simulink model "mod_integrador"  (R2020a)
settings: Solver=FixedStepAuto  StartTime=0.0  StopTime=t_fim  FixedStep=dt_sim  RelTol=1e-3
values from neighbouring files (symbols this model uses):
  Ac = [0, 1;0, 0]    [init.m]    (also in run.m = evalin('base', 'Ac'))
  Bc = [0; 1]    [init.m]    (also in run.m = evalin('base', 'Bc'))
  bf = aux(:,end)    [matrizes_ss_mpc_dualmode_switching.m]    (also in run.m = evalin('base', 'bf'))
  cbar = repmat(c,Np,1)    [matrizes_ss_mpc_dualmode_switching.m]    (also in run.m = evalin('base', 'cbar'))
  dt_sim = 0.001    [init.m]
  H = zeros(n*Np,p*Np)    [matrizes_ss_mpc_dualmode_switching.m]    (also in run.m = evalin('base', 'H'))
  Hf = H(end-n+1:end,:)    [matrizes_ss_mpc_dualmode_switching.m]    (also in run.m = evalin('base', 'Hf'))
  Lbar = blkdiag(Lbar,L)    [matrizes_ss_mpc_dualmode_switching.m]    (also in run.m = evalin('base', 'Lbar'))
  p = find(dt == 1, 2, 'last')    [get_xr.m]    (also in init.m = N - 1; matrizes_ss_mpc_dualmode_switching.m = size(Gamma,2); run.m = evalin('base', 'p'))
  Pf = dlyap(Phib',Phib'*Q*Phib + K'*R*K)    [matrizes_ss_mpc_dualmode_switching.m]    (also in run.m = evalin('base', 'Pf'))
  Phi1Np = [Phi1Np;Phi^i]    [matrizes_ss_mpc_dualmode_switching.m]    (also in run.m = evalin('base', 'Phi1Np'))
  PhiNp = Phi^Np    [matrizes_ss_mpc_dualmode_switching.m]    (also in run.m = evalin('base', 'PhiNp'))
  Qbar = blkdiag(Qbar,Q)    [matrizes_ss_mpc_dualmode_switching.m]    (also in run.m = evalin('base', 'Qbar'))
  Rbar = blkdiag(Rbar,R)    [matrizes_ss_mpc_dualmode_switching.m]    (also in run.m = evalin('base', 'Rbar'))
  Sf = aux(:,1:(end-1))    [matrizes_ss_mpc_dualmode_switching.m]    (also in run.m = evalin('base', 'Sf'))
  T = sum(dtr)    [init.m]
  tr = [2, 3, 5, 6]'    [init.m]    (also in run.m = evalin('base', 'tr'))
  ur = [1, 0, -1, 0]'    [init.m]    (also in run.m = evalin('base', 'ur'))
  x0 = [-0.5; -1]    [init.m]    (also in mpc_dualmode_switching.m = zeros(size(fqp, 1), 1); run.m = y_(end,:)')
  x_target = x0    [init.m]    (also in run.m)
settings Model: Creator=Daniel  LastModifiedBy=Daniel
settings DataIOCC: SaveOutput=off  DSMLogging=off  SaveTime=off

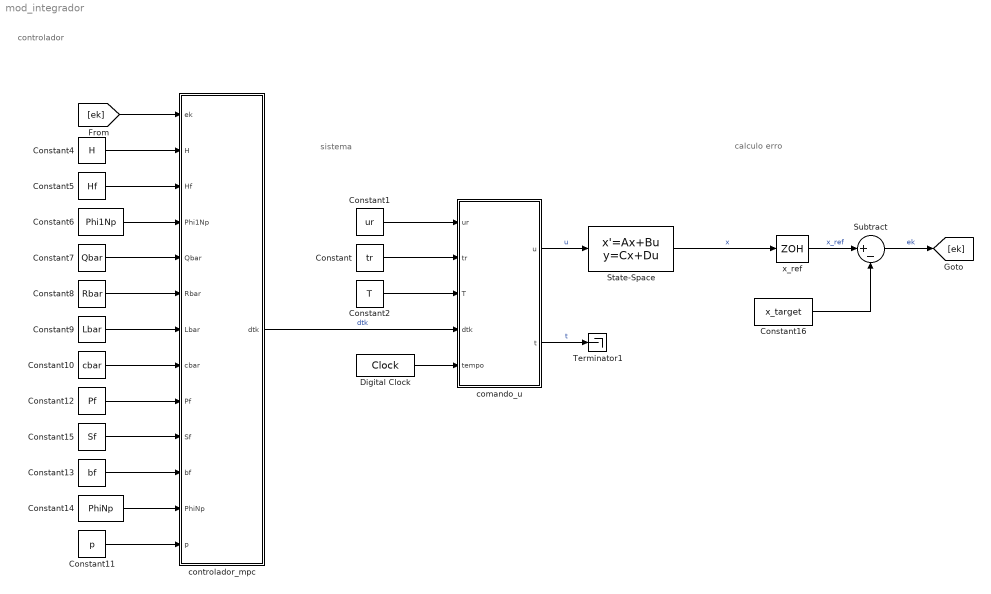
== system mod_integrador ==
  note: calculo erro
  note: controlador
  note: sistema
  Constant : Constant  Value=tr
  Constant1 : Constant  Value=ur
  Constant10 : Constant  Value=cbar
  Constant11 : Constant  Value=p
  Constant12 : Constant  Value=Pf
  Constant13 : Constant  Value=bf
  Constant14 : Constant  Value=PhiNp
  Constant15 : Constant  Value=Sf
  Constant16 : Constant  Value=x_target
  Constant2 : Constant  Value=T
  Constant4 : Constant  Value=H
  Constant5 : Constant  Value=Hf
  Constant6 : Constant  Value=Phi1Np
  Constant7 : Constant  Value=Qbar
  Constant8 : Constant  Value=Rbar
  Constant9 : Constant  Value=Lbar
  Digital Clock : DigitalClock  SampleTime=dt_sim
  State-Space : StateSpace  A=Ac  B=Bc  C=eye(2)  D=[0;0]  InitialCondition=x0
  Subtract : Sum  Inputs=|+-
  Terminator1 : Terminator
  comando_u : MATLAB Function  TreatAsAtomicUnit=on
  controlador_mpc : MATLAB Function  TreatAsAtomicUnit=on
  x_ref : ZeroOrderHold  SampleTime=T
  wires:
  State-Space/1 -> x_ref/1  "x"
  comando_u/1(u) -> State-Space/1  "u"
  Constant1/1 -> comando_u/1(ur)
  Constant/1 -> comando_u/2(tr)
  Digital Clock/1 -> comando_u/5(tempo)
  comando_u/2(t) -> Terminator1/1  "t"
  Constant2/1 -> comando_u/3(T)
  x_ref/1 -> Subtract/1  "x_ref"
  Constant11/1 -> controlador_mpc/13(p)
  [ek] -> controlador_mpc/1(ek)
  Constant4/1 -> controlador_mpc/2(H)
  Constant5/1 -> controlador_mpc/3(Hf)
  Constant6/1 -> controlador_mpc/4(Phi1Np)
  Constant14/1 -> controlador_mpc/12(PhiNp)
  Constant12/1 -> controlador_mpc/9(Pf)
  Constant13/1 -> controlador_mpc/11(bf)
  Constant7/1 -> controlador_mpc/5(Qbar)
  Constant8/1 -> controlador_mpc/6(Rbar)
  Constant9/1 -> controlador_mpc/7(Lbar)
  Constant10/1 -> controlador_mpc/8(cbar)
  Constant15/1 -> controlador_mpc/10(Sf)
  Constant16/1 -> Subtract/2
  Subtract/1 -> [ek]  "ek"
  controlador_mpc/1(dtk) -> comando_u/4(dtk)  "dtk"

== matlab function mod_integrador/controlador_mpc ==
  settings: updateMethod=DISCRETE  sampleTime=T
  data: ek input; dtk output; H input; Hf input; Phi1Np input; Qbar input; Rbar input; Lbar input; cbar input; Pf input; Sf input; bf input; PhiNp input; p input
function dtk = fcn(ek,H,Hf,Phi1Np,Qbar,Rbar,Lbar,cbar,Pf,Sf,bf,PhiNp,p)
    
    dtk_ = mpc_dualmode_switching(ek,H,Hf,Phi1Np,Qbar,Rbar,Lbar,cbar,Pf,Sf,bf,PhiNp,p);
    dtk  = dtk_(1:3);

== matlab function mod_integrador/comando_u ==
  data: ur input; tr input; T input; dtk input; u output; tempo input; t output
function [u,t] = fcn(ur, tr, T, dtk, tempo)
    
    [u,t] = fn_comando_u(ur, tr, T, dtk, tempo);
